simulink model "LA_input_generator"  (R2022a)
settings: Solver=VariableStepAuto  StartTime=0.0  StopTime=100  RelTol=1e-3
undefined symbols (not defined in the file): Arm_resistance, C, D, h, J, Ke, Km, Ks, Kt, La, M_load, M_screw
settings Model: Creator=royka  LastModifiedBy=royka
settings DataIOCC: ExternalInput=tt  LoadExternalInput=on

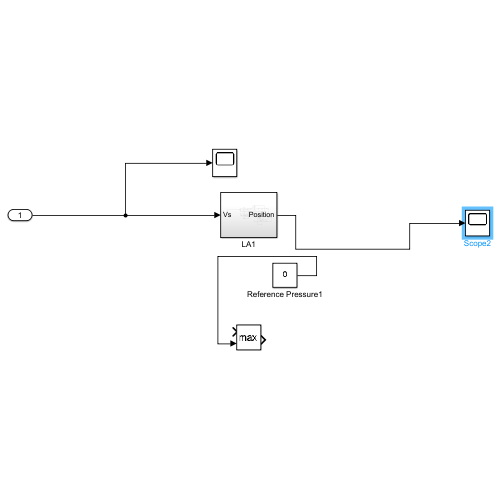
[thumbnail: Simulink's stored preview of the top-level diagram]
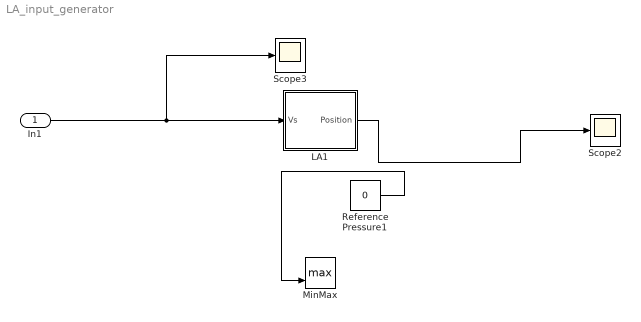
== system LA_input_generator ==
  In1 : Inport
  LA1 : Subsystem
  MinMax : MinMax  Function=max  Inputs=2
  Reference Pressure1 : Constant  Value=0
  Scope2 : Scope
  Scope3 : Scope
  wires:
  In1/1 -> Scope3/1, LA1/1(Vs)
  LA1/1(Position) -> Scope2/1
  Reference Pressure1/1 -> MinMax/2

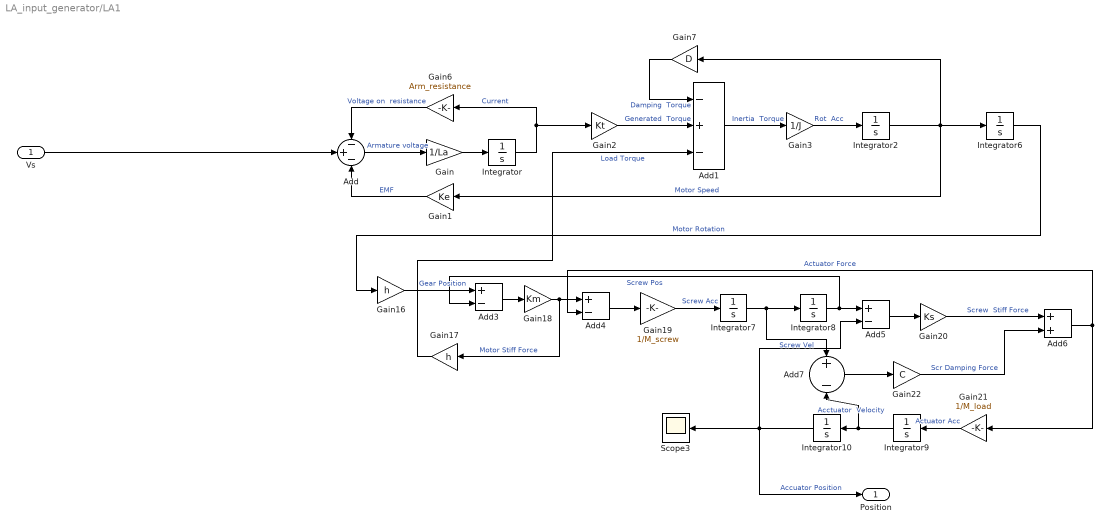
== system LA_input_generator/LA1 ==
  Vs : Inport
  Add : Sum  Inputs=-+-
  Add1 : Sum  Inputs=-+-
  Add{3..5,7} (4 alike) : Sum  Inputs=+-
  Add6 : Sum
  Gain : Gain  Gain=1/La
  Gain1 : Gain  Gain=Ke
  Gain16 : Gain  Gain=h
  Gain17 : Gain  Gain=h
  Gain18 : Gain  Gain=Km
  Gain19 : Gain  Gain=1/M_screw
  Gain2 : Gain  Gain=Kt
  Gain20 : Gain  Gain=Ks
  Gain21 : Gain  Gain=1/M_load
  Gain22 : Gain  Gain=C
  Gain3 : Gain  Gain=1/J
  Gain6 : Gain  Gain=Arm_resistance
  Gain7 : Gain  Gain=D
  Integrator{,2,6..10} (7 alike) : Integrator
  Scope3 : Scope
  Position : Outport
  wires:
  Gain16/1 -> Add3/1  "Gear Position"
  Gain/1 -> Integrator/1
  Integrator8/1 -> Add3/2, Add5/1  "Screw Pos"
  Gain19/1 -> Integrator7/1  "Screw Acc"
  Gain2/1 -> Add1/2  "Generated  Torque"
  Gain20/1 -> Add6/1  "Screw  Stiff Force"
  Add1/1 -> Gain3/1  "Inertia  Torque"
  Vs/1 -> Add/2
  Gain17/1 -> Add1/3  "Load Torque"
  Gain1/1 -> Add/3  "EMF"
  Gain21/1 -> Integrator9/1  "Actuator Acc"
  Add/1 -> Gain/1  "Armature voltage"
  Add3/1 -> Gain18/1
  Gain22/1 -> Add6/2  "Scr Damping Force"
  Integrator9/1 -> Add7/2, Integrator10/1  "Acctuator  Velocity"
  Add7/1 -> Gain22/1
  Add5/1 -> Gain20/1
  Integrator/1 -> Gain6/1, Gain2/1  "Current"
  Gain6/1 -> Add/1  "Voltage on  resistance"
  Gain3/1 -> Integrator2/1  "Rot  Acc"
  Add6/1 -> Gain21/1, Add4/2  "Actuator Force"
  Integrator10/1 -> Position/1, Add5/2, Scope3/1  "Accuator Position"
  Add4/1 -> Gain19/1
  Integrator2/1 -> Gain1/1, Integrator6/1, Gain7/1  "Motor Speed"
  Integrator6/1 -> Gain16/1  "Motor Rotation"
  Gain7/1 -> Add1/1  "Damping  Torque"
  Integrator7/1 -> Add7/1, Integrator8/1  "Screw Vel"
  Gain18/1 -> Gain17/1, Add4/1  "Motor Stiff Force"
